simulink model "MOSSE_HDL_HIL_final"  (Simulink 8.1)
settings: Solver=FixedStepDiscrete  SolverMode=SingleTasking  StartTime=0.0  StopTime=20*30*640*360  RelTol=1e-3
InitFcn:
  | %% DSPBuilder Start
  | alt_dspbuilder_update_model(bdroot)
  | %% DSPBuilder End
  | K_shift = 4
  | 
  | ksize = 5
  | load('Gauss_coeff.mat')
  | tic
StopFcn:
  | % r = rcount.Data(:,:);
  | % w = wcount.Data(:,:);
  | % d = dout.Data(:,:);
  | % ir = read.Data(:,:);
  | % iw = write.Data(:,:);
  | % z = double([ir iw d r w]');
  | %logic_analyzer
  | toc
undefined symbols (not defined in the file or in its folder): gray, psr, source_1, source_2, State_Machine, State_Transition_Table1
libraries: allblocks_alteradspbuilder2 x75, hdldemolib x2, dspsigattribs x2, dspmtrx3 x2, visionsinks x1, visiontextngfix x1, dspvision x1
(part 2 of 2)

== stateflow chart Video_TestBench1/Write_control_subsys/Write_control_STM ==
  settings: executeAtInitialization=1
  state state2
    % Автомат управления сигналом записи кадра в память
    entry:
    x_coord = x;
    y_coord = y;
    enable_write = false;
    to_workspace_enable = false;
  state state1
    % Условия по-умолчанию
    entry:
    enable_write = false;
    x_coord = fi(0,0,10,0);
    y_coord = fi(0,0,9,0);
    frame_num = uint16(0);
    to_workspace_enable = false;
  state state3
    entry:
    enable_write = true;
  state state4
    entry:
    enable_write = false;
  state state5
    % Кадр записан
    % Обновление значений смещения
    entry:
    enable_write = false;
  state state6
    % Обновление значений координат
    entry:
    enable_write = false;
    frame_num = frame_count;
    to_workspace_enable = true;
  state1 -> (junction 106) [order 2]
  (default) -> state1
  (junction 106) -> state1
  state1 -> state2 [order 1] : {count = fi(0,0,8,0);
      | frame_count = uint16(0);
      | x = fi(x_init,0,10,0);
      | y = fi(y_init,0,9,0);
      | temp_x = fi(x + 128,0,10,0);
      | temp_y = fi(y + count,0,9,0);
      | Dx = int8(0);
      | Dy = int8(0);}
  state2 -> (junction 107) [order 3]
  (junction 107) -> state2
  (junction 108) -> state2
  state2 -> (junction 109) [order 2] : [comp_shift_finish == true && count == 0]
  (junction 111) -> (junction 108)
  (junction 109) -> (junction 113)
  state2 -> state3 [order 1] : [addr_x == x && addr_y == temp_y && comp_shift_finish == false]
  state3 -> (junction 110) [order 1] : [addr_x ~= temp_x]
  (junction 110) -> state3
  state3 -> state4 [order 2] : {count = fi(count + 1,0,8,0);
      | temp_y = fi(y + count,0,9,0);}
  state4 -> (junction 111) [order 1] : [count ~= 128]
  (junction 115) -> (junction 111)
  state4 -> state5 [order 2] : {count = fi(0,0,8,0);
      | frame_count = uint16(frame_count + 1);}
  state5 -> (junction 112) [order 2]
  (junction 112) -> state5
  (junction 113) -> state5
  state5 -> state6 [order 1] : {Dx = dx;
      | Dy = dy;}
  state6 -> (junction 114) [order 2]
  (junction 114) -> state6
  state6 -> (junction 115) [order 1] : {x = fi(x + Dx,0,10,0);
      | y = fi(y + Dy,0,9,0);
      | temp_x = fi(x + 128,0,10,0);
      | temp_y = fi(y + count,0,9,0);}
  (junction 116) -> state6
  data: x_coord output fixdt(0,10,0); y_coord output fixdt(0,9,0); addr_x input fixdt(0,10,0); count local fixdt(0,8,0); x local fixdt(0,10,0); addr_y input fixdt(0,9,0); y local fixdt(0,9,0); dx input int8; dy input int8; Dx local int8; Dy local int8; temp_x local fixdt(0,10,0); temp_y local fixdt(0,9,0); enable_write output boolean; comp_shift_finish input boolean; to_workspace_enable output boolean; x_init input uint16; y_init input uint16; frame_count local uint16; frame_num output uint16; enable_tracking input boolean

== matlab function Video_TestBench1/Transpone Counter ==
  data: X output fixdt(0,10,0); clear input boolean; en input boolean; Y output fixdt(0,9,0)
function [X, Y]  = count(clear, en)

%result_nt = numerictype(0,12,0);
col_nt = numerictype(0,10,0);
row_nt = numerictype(0,9,0);

result_fm = fimath('OverflowMode', 'saturate', 'RoundMode', 'floor');
m = fi(640, 0,10,0, result_fm);
n = fi(360, 0,9,0, result_fm);
% persistent count_reg 
persistent column row

% if isempty(count_reg)
%     count_reg = fi(0, result_nt, result_fm);
% end

if isempty(column)
    column = fi(0, col_nt, result_fm);
end

if isempty(row)
    row = fi(0, row_nt, result_fm);
end

if clear
    row = fi(0, row_nt, result_fm);
    column = fi(0, col_nt, result_fm);
    % count_reg = fi(0, result_nt, result_fm);
elseif en
     
     if (column == (m-1))
         if(row ~= (n-1))
             inc_r = row + fi(1, row_nt, result_fm);
             row = fi(inc_r, row_nt, result_fm);
         else row = fi(0, row_nt, result_fm);
             
         end
         column = fi(0, col_nt, result_fm);
     else
         inc_c = column + fi(1, col_nt, result_fm);
         column = fi(inc_c, col_nt, result_fm);
     end
     %count_reg = fi(column*n + row, result_nt, result_fm);
end

X = column;
Y = row;
% count = count_reg;

end
